simulink model "PIL_Arduino_v04_r2018a"  (R2019a)
settings: Solver=VariableStepAuto  StartTime=0.0  StopTime=Tsim  RelTol=1e-3
values from neighbouring files (symbols this model uses):
  Ac = [[1 0] ... (first row only)    [main_PIL_Arduino_v04.m]    (also in result_data.mat = [1  0; 1  1])
  Bc = [1 0]'    [main_PIL_Arduino_v04.m]    (also in result_data.mat = [1 0])
  Cc = [1 0]    [main_PIL_Arduino_v04.m]    (also in result_data.mat)
  Ts = 1/fs    (= 0.030303030303)    [main_PIL_Arduino_v04.m]    (also in result_data.mat)
  xo = [-1 1]'    [main_PIL_Arduino_v04.m]    (also in result_data.mat = [-1 1])
undefined symbols (not defined in the file or in its folder): serial
libraries: instrumentlib x3
settings Model: EnablePacing=on  Creator=ricardo  LastModifiedBy=Ricardo
settings DataIOCC: ReturnWorkspaceOutputs=off
settings DebuggingCC: ArithmeticOperatorsInVariantConditions=warning

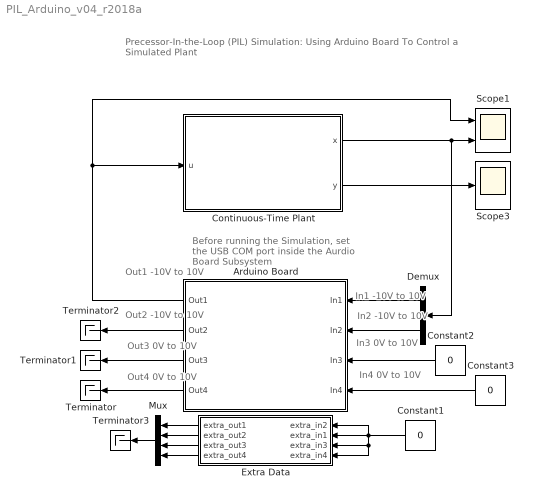
== system PIL_Arduino_v04_r2018a ==
  note: Out1
      | -10V to 10V
  note: Precessor-In-the-Loop (PIL) Simulation:
      | Using Arduino Board To Control a Simulated Plant
  note: Out2
      | -10V to 10V
  note: Out3
      | 0V to 10V
  note: Out4
      | 0V to 10V
  note: In1
      | -10V to 10V
  note: In2
      | -10V to 10V
  note: In3
      | 0V to 10V
  note: In4
      | 0V to 10V
  note: Before running the Simulation, set the USB COM port inside the Aurdio Board Subsystem
  Arduino Board : Subsystem
      mask Display: image('UTS_MKR_Board_v03.png')
  Constant1 : Constant  Value=0
  Constant2 : Constant  Value=0
  Constant3 : Constant  Value=0
  Continuous-Time Plant : Subsystem
  Demux : Demux  Outputs=2
  Extra Data : Subsystem
  Mux : Mux
  Scope1 : Scope  NumInputPorts=2
  Scope3 : Scope
  Terminator{,1..3} (4 alike) : Terminator
  wires:
  Continuous-Time Plant/2(y) -> Scope3/1
  Continuous-Time Plant/1(x) -> Scope1/2, Demux/1
  Demux/1 -> Arduino Board/1(In1)
  Demux/2 -> Arduino Board/2(In2)
  Arduino Board/1(Out1) -> Scope1/1, Continuous-Time Plant/1(u)
  Arduino Board/2(Out2) -> Terminator2/1
  Arduino Board/3(Out3) -> Terminator1/1
  Arduino Board/4(Out4) -> Terminator/1
  Constant2/1 -> Arduino Board/3(In3)
  Constant3/1 -> Arduino Board/4(In4)
  Constant1/1 -> Extra Data/4(extra_in4), Extra Data/3(extra_in3), Extra Data/2(extra_in1), Extra Data/1(extra_in2)
  Extra Data/1(extra_out1) -> Mux/1
  Extra Data/2(extra_out2) -> Mux/2
  Extra Data/3(extra_out3) -> Mux/3
  Extra Data/4(extra_out4) -> Mux/4
  Mux/1 -> Terminator3/1

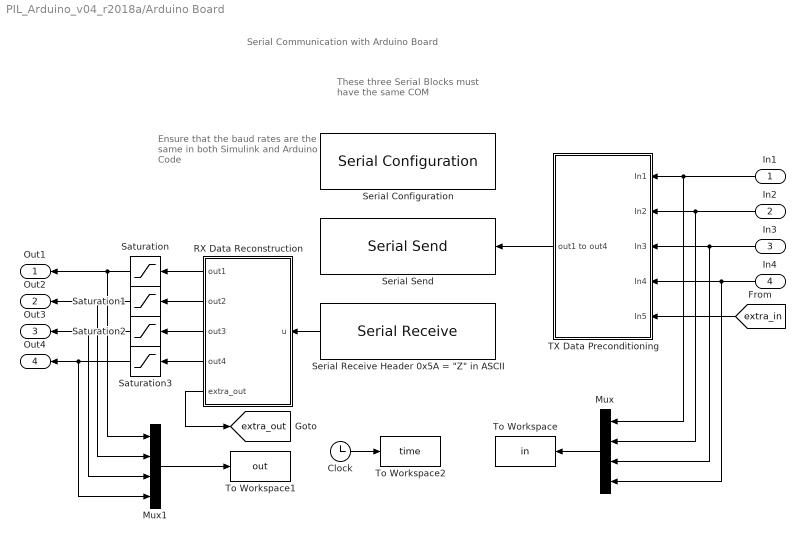
== system PIL_Arduino_v04_r2018a/Arduino Board ==
  note: Ensure that the baud rates are the same in both Simulink and Arduino Code
  note: Serial Communication with Arduino Board
  note: These three Serial Blocks must have the same COM
  In1 : Inport
  In2 : Inport  Port=2
  In3 : Inport  Port=3
  In4 : Inport  Port=4
  Clock : Clock
  Mux : Mux
  Mux1 : Mux
  RX Data Reconstruction : MATLAB Function  TreatAsAtomicUnit=on
  Saturation : Saturate  UpperLimit=10  LowerLimit=-10
  Saturation1 : Saturate  UpperLimit=10  LowerLimit=-10
  Saturation2 : Saturate  UpperLimit=10  LowerLimit=0
  Saturation3 : Saturate  UpperLimit=10  LowerLimit=0
  Serial Configuration : instrumentlib/Serial Configuration  Priority=-200000  ComPortMenu=/dev/cu.usbmodem14101  ComPort=/dev/cu.usbmodem14101  ObjConstructor=serial('/dev/cu.usbmodem14101');  BaudRate=115200  DataBits=8  Parity=none  StopBits=1  FlowControl=none  Timeout=0.0001  ByteOrder=LittleEndian
  "Serial Receive Header 0x5A = \"Z\" in ASCII" : instrumentlib/Serial Receive  ComPortMenu=<Please select a port...>  ComPort=/dev/cu.usbmodem14101  ObjConstructor=serial('/dev/tty.usbmodem14601');  Header=Z  Terminator=<none>  DataSize=8  DataType=uint8  EnableBlockingMode=on  ActionDataUnavailable=Output last received value  CustomValue=0  SampleTime=0.5*Ts
  Serial Send : instrumentlib/Serial Send  ComPortMenu=/dev/cu.usbmodem14101  ComPort=/dev/cu.usbmodem14101  ObjConstructor=serial('/dev/cu.usbmodem14101');  Terminator=<none>  EnableBlockingMode=on
  TX Data Preconditioning : Subsystem
  To Workspace : ToWorkspace  VariableName=in  SampleTime=-1
  To Workspace1 : ToWorkspace  VariableName=out  SampleTime=-1
  To Workspace2 : ToWorkspace  VariableName=time  SampleTime=-1
  Out1 : Outport  VectorParamsAs1DForOutWhenUnconnected=off
  Out2 : Outport  Port=2  VectorParamsAs1DForOutWhenUnconnected=off
  Out3 : Outport  Port=3  VectorParamsAs1DForOutWhenUnconnected=off
  Out4 : Outport  Port=4  VectorParamsAs1DForOutWhenUnconnected=off
  tag scope: extra_out=global
  wires:
  "Serial Receive Header 0x5A = \"Z\" in ASCII"/1 -> RX Data Reconstruction/1(u)
  In1/1 -> TX Data Preconditioning/1(In1), Mux/1
  In2/1 -> TX Data Preconditioning/2(In2), Mux/2
  In3/1 -> TX Data Preconditioning/3(In3), Mux/3
  In4/1 -> TX Data Preconditioning/4(In4), Mux/4
  TX Data Preconditioning/1(out1 to out4) -> Serial Send/1
  RX Data Reconstruction/1(out1) -> Saturation/1
  RX Data Reconstruction/2(out2) -> Saturation1/1
  RX Data Reconstruction/3(out3) -> Saturation2/1
  Mux/1 -> To Workspace/1
  Mux1/1 -> To Workspace1/1
  Clock/1 -> To Workspace2/1
  Saturation/1 -> Out1/1, Mux1/1
  Saturation1/1 -> Out2/1, Mux1/2
  Saturation2/1 -> Out3/1, Mux1/3
  Saturation3/1 -> Out4/1, Mux1/4
  RX Data Reconstruction/4(out4) -> Saturation3/1
  [extra_in] -> TX Data Preconditioning/5(In5)
  RX Data Reconstruction/5(extra_out) -> [extra_out]

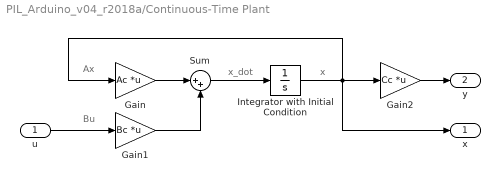
== system PIL_Arduino_v04_r2018a/Continuous-Time Plant ==
  note: x
  note: x_dot
  note: Bu
  note: Ax
  u : Inport
  Gain : Gain  Gain=Ac  Multiplication=Matrix(K*u)
  Gain1 : Gain  Gain=Bc  Multiplication=Matrix(K*u)
  Gain2 : Gain  Gain=Cc  Multiplication=Matrix(K*u)
  Integrator with Initial Condition : Integrator  InitialCondition=xo
  Sum : Sum  Inputs=|++
  x : Outport  VectorParamsAs1DForOutWhenUnconnected=off
  y : Outport  Port=2  VectorParamsAs1DForOutWhenUnconnected=off
  wires:
  u/1 -> Gain1/1
  Gain1/1 -> Sum/2
  Sum/1 -> Integrator with Initial Condition/1
  Gain/1 -> Sum/1
  Integrator with Initial Condition/1 -> Gain2/1, x/1, Gain/1
  Gain2/1 -> y/1

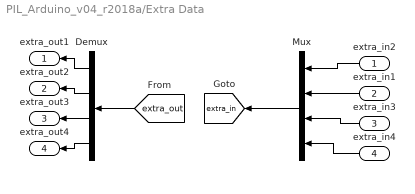
== system PIL_Arduino_v04_r2018a/Extra Data ==
  extra_in2 : Inport
  extra_in1 : Inport  Port=2
  extra_in3 : Inport  Port=3
  extra_in4 : Inport  Port=4
  Demux : Demux
  Mux : Mux
  extra_out1 : Outport
  extra_out2 : Outport  Port=2
  extra_out3 : Outport  Port=3
  extra_out4 : Outport  Port=4
  tag scope: extra_in=global
  wires:
  extra_in4/1 -> Mux/4
  extra_in3/1 -> Mux/3
  extra_in1/1 -> Mux/2
  extra_in2/1 -> Mux/1
  Mux/1 -> [extra_in]
  [extra_out] -> Demux/1
  Demux/1 -> extra_out1/1
  Demux/2 -> extra_out2/1
  Demux/3 -> extra_out3/1
  Demux/4 -> extra_out4/1

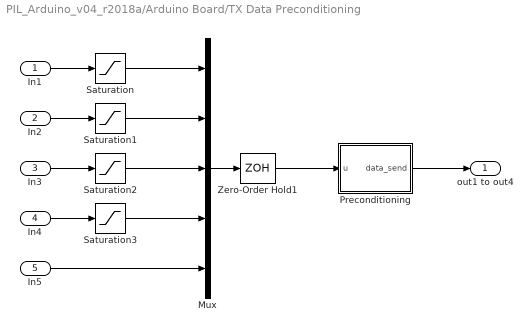
== system PIL_Arduino_v04_r2018a/Arduino Board/TX Data Preconditioning ==
  In1 : Inport
  In2 : Inport  Port=2
  In3 : Inport  Port=3
  In4 : Inport  Port=4
  In5 : Inport  Port=5
  Mux : Mux  Inputs=5
  Preconditioning : MATLAB Function  TreatAsAtomicUnit=on
  Saturation : Saturate  UpperLimit=10  LowerLimit=-10
  Saturation1 : Saturate  UpperLimit=10  LowerLimit=-10
  Saturation2 : Saturate  UpperLimit=10  LowerLimit=0
  Saturation3 : Saturate  UpperLimit=10  LowerLimit=0
  Zero-Order Hold1 : ZeroOrderHold  SampleTime=Ts
  out1 to out4 : Outport  VectorParamsAs1DForOutWhenUnconnected=off
  wires:
  In1/1 -> Saturation/1
  Preconditioning/1(data_send) -> out1 to out4/1
  Saturation3/1 -> Mux/4
  Saturation2/1 -> Mux/3
  Saturation1/1 -> Mux/2
  In2/1 -> Saturation1/1
  Mux/1 -> Zero-Order Hold1/1
  In4/1 -> Saturation3/1
  In3/1 -> Saturation2/1
  Saturation/1 -> Mux/1
  Zero-Order Hold1/1 -> Preconditioning/1(u)
  In5/1 -> Mux/5

== matlab function PIL_Arduino_v04_r2018a/Arduino Board/RX Data Reconstruction ==
  data: u input; out1 output; out2 output; out3 output; out4 output; extra_out output
function [out1, out2, out3, out4, extra_out] = fcn(u)
N_data=4;


out=zeros(N_data,1);
extra_out=zeros(4,1);

for k=1:N_data
    %% Reconstructing out1
    MSB_uint8 = u(2*k-1); % Least Significant Bits (8 bits)
    LSB_uint8 = u(2*k);  % Most Significant Bits (8 bits)

    % Transforming MSB_uint8 in 16 bits. 
    MSB_uint16 = uint16(MSB_uint8);     %  MSB_unit16 = 00000000 | MSB_uint8 
                                                          % MSB_uint8 is stored as LSB in MSB_uint16                                             
                                                          % Therefore, it has to be shifted in 8 positions

    MSB_uint16 =bitshift(MSB_uint16,8); % MSB_unit16 = MSB_uint8 | 00000000
    out1_uint16 = MSB_uint16+ uint16(LSB_uint8);  % out1_uint16 = MSB_uint8 | LSB_uint8

    %Finally, it is transformed in its original float number
    out(k) = double(out1_uint16)*0.001-10;  
end

out1 = out(1);
out2 = out(2);
out3 = out(3);
out4 = out(4);

== matlab function PIL_Arduino_v04_r2018a/Arduino Board/TX Data Preconditioning/Preconditioning ==
  data: u input; data_send output
function data_send = fcn(u)
N_data=4;

data_send=uint8(zeros(2*N_data+1,1));   % array of 2 bytes (2 variables of 8 bits) + Header

%Header
data_send(1)=hex2dec('AA');             %0xAA is for send data in this example

for k=1:N_data
    in = u(k);  %Input singal is between -10 to 10

    %% Data preconditioning to be transmitted as bytes

    in_pos = in+10; % to transform it in an unsigned signal between 0 to 20
    in_uint16= uint16(1000*in_pos); % Transforming it in an unsigned integer of 16 bits

    % Now, the 16 bits variable will be divided in 2 8bits variable.
    % in1_uint16 = MSB_uint8 | LSB_uint8
    % 255(dec) = 00000000|11111111 (16 bits)
    LSB_uint8  = uint8(bitand(in_uint16,255));   %Extraxting Least Significant Bits (8 bits)
    MSB_uint8 = uint8(bitshift(in_uint16,-8));    %Extraxting Most Significant Bits (8 bits)

    % Data is now put in an byte array to be transmitted
    data_send(2*k)=MSB_uint8;
    data_send(2*k+1)=LSB_uint8;
end
